simulink model "Test2Part3"  (R2024a)
settings: Solver=VariableStepDiscrete  StartTime=0.0  StopTime=1000  MaxStep=1  RelTol=1e-3
libraries: matrix_library x3
settings Model: Creator=katutu  LastModifiedBy=katutu

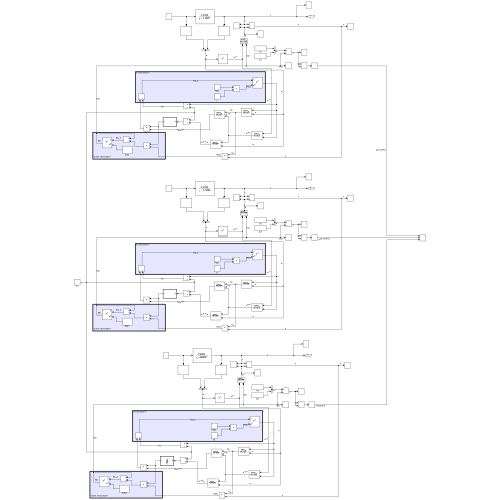
[thumbnail: Simulink's stored preview of the top-level diagram]
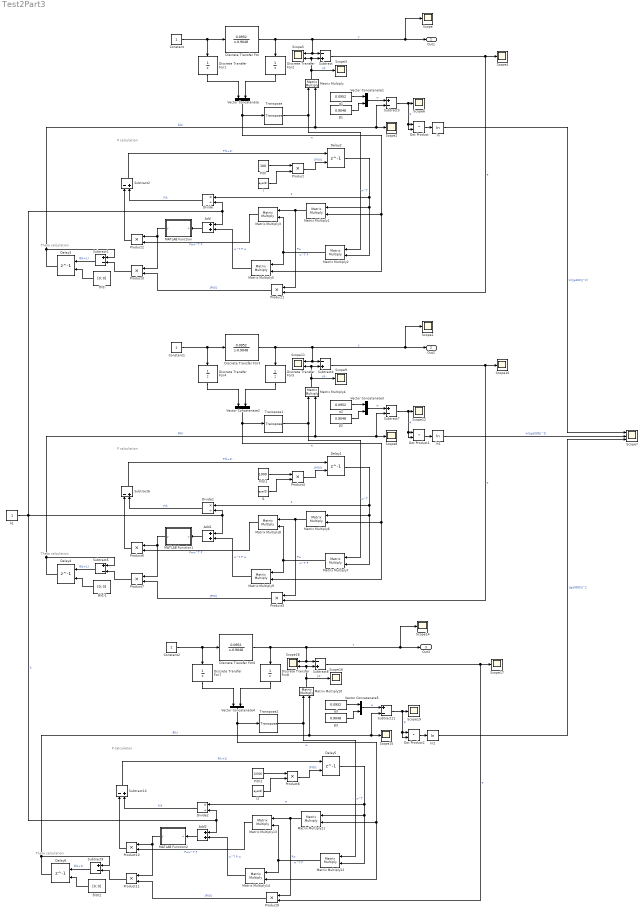
== system Test2Part3 ==
  note: P calculation
  note: Theta calculation
  note: Theta calculation
  note: P calculation
  note: Theta calculation
  note: P calculation
  Add : Sum
  Add1 : Sum
  Add2 : Sum
  Constant : Constant
  Constant1 : Constant
  Constant2 : Constant
  Delay{1..6} (6 alike) : Delay  DelayLength=1  InitialConditionSource=Input port  InitialCondition=0
      settings: InputPortMap=u0,p4
  Discrete Transfer Fcn : DiscreteTransferFcn  Numerator=[0.0952]  Denominator=[1 -0.9048]
  Discrete Transfer Fcn{1..2,4..5,7..8} (6 alike) : DiscreteTransferFcn  Denominator=[1 0]
  Discrete Transfer Fcn3 : DiscreteTransferFcn  Numerator=[0.0952]  Denominator=[1 -0.9048]
  Discrete Transfer Fcn6 : DiscreteTransferFcn  Numerator=[0.0952]  Denominator=[1 -0.9048]
  Divide : Product  Inputs=*/
  Divide1 : Product  Inputs=*/
  Divide2 : Product  Inputs=*/
  Dot Product : DotProduct  OutDataTypeStr=Inherit: Inherit via internal rule
  Dot Product1 : DotProduct  OutDataTypeStr=Inherit: Inherit via internal rule
  Dot Product2 : DotProduct  OutDataTypeStr=Inherit: Inherit via internal rule
  I : Constant  Value=eye(2)
  I1 : Constant  Value=eye(2)
  I2 : Constant  Value=eye(2)
  MATLAB Function : MATLAB Function  TreatAsAtomicUnit=on
  MATLAB Function1 : MATLAB Function  TreatAsAtomicUnit=on
  MATLAB Function2 : MATLAB Function  TreatAsAtomicUnit=on
  Matrix Multiply{,1..14} (15 alike) : Product  Multiplication=Matrix(*)
  P(0) : Constant  Value=100
  P(0)1 : Constant  Value=1000
  P(0)2 : Constant  Value=10000
  Product{,1..11} (12 alike) : Product
  Scope{,1..4,6,8..10,12,14..17,19} (15 alike) : Scope
  Scope11 : Scope  NumInputPorts=2
  Scope18 : Scope  NumInputPorts=2
  Scope5 : Scope  NumInputPorts=2
  Scope7 : Scope  NumInputPorts=3
  Subtract{,2,4,6,8,10} (6 alike) : Sum  Inputs=-+
  Subtract{1,3,5,7,9,11} (6 alike) : Sum  Inputs=+-
  Transpose : matrix_library/Transpose
  Transpose1 : matrix_library/Transpose
  Transpose2 : matrix_library/Transpose
  Vector Concatenate{,1..5} (6 alike) : Concatenate
  ln : Math  Operator=log
  ln1 : Math  Operator=log
  ln2 : Math  Operator=log
  α1 : Constant  Value=0.0952
  α2 : Constant  Value=0.0952
  α3 : Constant  Value=0.0952
  β1 : Constant  Value=0.9048
  β2 : Constant  Value=0.9048
  β3 : Constant  Value=0.9048
  θ(0) : Constant  Value=[0; 0]
  θ(0)1 : Constant  Value=[0; 0]
  θ(0)2 : Constant  Value=[0; 0]
  λ1 : Constant
  Out1 : Outport  SignalName=y
  Out2 : Outport  Port=2  SignalName=y
  Out3 : Outport  Port=3  SignalName=y
  wires:
  Constant/1 -> Discrete Transfer Fcn1/1, Discrete Transfer Fcn/1
  Discrete Transfer Fcn2/1 -> Vector Concatenate/2
  Discrete Transfer Fcn1/1 -> Vector Concatenate/1
  Vector Concatenate/1 -> Matrix Multiply5/2, Matrix Multiply1/2, Transpose/1  "w"
  Matrix Multiply/1 -> Subtract/2, Scope5/2, Scope3/1  "yp"
  Subtract/1 -> Scope4/1, Product1/2  "e"
  Transpose/1 -> Matrix Multiply2/1, Matrix Multiply/1  "w^T"
  Delay3/1 -> Matrix Multiply/2, Subtract3/2, Scope2/1, Subtract1/1  "θ(k)"
  Discrete Transfer Fcn/1 -> Out1/1, Scope/1, Scope5/1, Subtract/1, Discrete Transfer Fcn2/1  "y"
  λ1/1 -> Divide/2, Add/1, Add1/1, Divide1/2, Divide2/2, Add2/1  "λ"
  Delay2/1 -> Divide/1, Matrix Multiply2/2, Matrix Multiply1/1  "P"
  I/1 -> Product/2
  Product/1 -> Delay2/2  "[P(0)]"
  Matrix Multiply1/1 -> Product1/1, Matrix Multiply3/1  "Pw"
  Matrix Multiply2/1 -> Matrix Multiply3/2, Matrix Multiply5/1  "w^T P"
  Matrix Multiply3/1 -> Product2/2  "Pww^T P"
  MATLAB Function/1(y) -> Product3/1, Product2/1
  Add/1 -> MATLAB Function/1(u)
  Matrix Multiply5/1 -> Add/2  "w^T P w"
  P(0)/1 -> Product/1
  Divide/1 -> Subtract2/2  "P/λ"
  Product2/1 -> Subtract2/1
  Subtract2/1 -> Delay2/1  "P(k+1)"
  θ(0)/1 -> Delay3/2
  Subtract1/1 -> Delay3/1  "θ(k+1)"
  Product1/1 -> Product3/2  "[P(0)]"
  Product3/1 -> Subtract1/2
  α1/1 -> Vector Concatenate1/1
  β1/1 -> Vector Concatenate1/2
  Vector Concatenate1/1 -> Subtract3/1  "w"
  Subtract3/1 -> Dot Product/2, Dot Product/1, Scope6/1  "φ"
  Dot Product/1 -> ln/1
  ln/1 -> Scope7/1  "ln(||φ100||^2)"
  Discrete Transfer Fcn3/1 -> Out2/1, Scope1/1, Scope11/1, Subtract4/1, Discrete Transfer Fcn5/1  "y"
  I1/1 -> Product4/2
  Vector Concatenate2/1 -> Matrix Multiply9/2, Matrix Multiply6/2, Transpose1/1  "w"
  Product4/1 -> Delay1/2  "[P(0)]"
  Discrete Transfer Fcn4/1 -> Vector Concatenate2/1
  Delay4/1 -> Matrix Multiply4/2, Subtract7/2, Scope8/1, Subtract5/1  "θ(k)"
  Delay1/1 -> Divide1/1, Matrix Multiply7/2, Matrix Multiply6/1  "P"
  MATLAB Function1/1(y) -> Product7/1, Product6/1
  Matrix Multiply6/1 -> Product5/1, Matrix Multiply8/1  "Pw"
  θ(0)1/1 -> Delay4/2
  Matrix Multiply4/1 -> Subtract4/2, Scope11/2, Scope9/1  "yp"
  Transpose1/1 -> Matrix Multiply7/1, Matrix Multiply4/1  "w^T"
  Subtract7/1 -> Dot Product1/2, Dot Product1/1, Scope12/1  "φ"
  Matrix Multiply7/1 -> Matrix Multiply8/2, Matrix Multiply9/1  "w^T P"
  Product7/1 -> Subtract5/2
  Constant1/1 -> Discrete Transfer Fcn4/1, Discrete Transfer Fcn3/1
  Vector Concatenate3/1 -> Subtract7/1  "w"
  Discrete Transfer Fcn5/1 -> Vector Concatenate2/2
  Add1/1 -> MATLAB Function1/1(u)
  P(0)1/1 -> Product4/1
  Matrix Multiply9/1 -> Add1/2  "w^T P w"
  Product5/1 -> Product7/2  "[P(0)]"
  Matrix Multiply8/1 -> Product6/2  "Pww^T P"
  Subtract6/1 -> Delay1/1  "P(k+1)"
  Subtract5/1 -> Delay4/1  "θ(k+1)"
  β2/1 -> Vector Concatenate3/2
  Subtract4/1 -> Scope10/1, Product5/2  "e"
  ln1/1 -> Scope7/2  "ln(||φ1000||^2)"
  α2/1 -> Vector Concatenate3/1
  Product6/1 -> Subtract6/1
  Divide1/1 -> Subtract6/2  "P/λ"
  Dot Product1/1 -> ln1/1
  Discrete Transfer Fcn6/1 -> Out3/1, Scope14/1, Scope18/1, Subtract8/1, Discrete Transfer Fcn8/1  "y"
  I2/1 -> Product8/2
  Vector Concatenate4/1 -> Matrix Multiply14/2, Matrix Multiply11/2, Transpose2/1  "w"
  Product8/1 -> Delay5/2  "[P(0)]"
  Discrete Transfer Fcn7/1 -> Vector Concatenate4/1
  Delay6/1 -> Matrix Multiply10/2, Subtract11/2, Scope15/1, Subtract9/1  "θ(k)"
  Delay5/1 -> Divide2/1, Matrix Multiply12/2, Matrix Multiply11/1  "P"
  MATLAB Function2/1(y) -> Product11/1, Product10/1
  Matrix Multiply11/1 -> Product9/1, Matrix Multiply13/1  "Pw"
  θ(0)2/1 -> Delay6/2
  Matrix Multiply10/1 -> Subtract8/2, Scope18/2, Scope16/1  "yp"
  Transpose2/1 -> Matrix Multiply12/1, Matrix Multiply10/1  "w^T"
  Subtract11/1 -> Dot Product2/2, Dot Product2/1, Scope19/1  "φ"
  Matrix Multiply12/1 -> Matrix Multiply13/2, Matrix Multiply14/1  "w^T P"
  Product11/1 -> Subtract9/2
  Constant2/1 -> Discrete Transfer Fcn7/1, Discrete Transfer Fcn6/1
  Vector Concatenate5/1 -> Subtract11/1  "w"
  Discrete Transfer Fcn8/1 -> Vector Concatenate4/2
  Add2/1 -> MATLAB Function2/1(u)
  P(0)2/1 -> Product8/1
  Matrix Multiply14/1 -> Add2/2  "w^T P w"
  Product9/1 -> Product11/2  "[P(0)]"
  Matrix Multiply13/1 -> Product10/2  "Pww^T P"
  Subtract10/1 -> Delay5/1  "P(k+1)"
  Subtract9/1 -> Delay6/1  "θ(k+1)"
  β3/1 -> Vector Concatenate5/2
  Subtract8/1 -> Scope17/1, Product9/2  "e"
  ln2/1 -> Scope7/3  "||φ10000||^2"
  α3/1 -> Vector Concatenate5/1
  Product10/1 -> Subtract10/1
  Divide2/1 -> Subtract10/2  "P/λ"
  Dot Product2/1 -> ln2/1

== matlab function Test2Part3/MATLAB Function ==
  data: u input; y output
function y = fcn(u)

y = inv(u);

== matlab function Test2Part3/MATLAB Function2 ==
  data: u input; y output
function y = fcn(u)

y = inv(u);

== matlab function Test2Part3/MATLAB Function1 ==
  data: u input; y output
function y = fcn(u)

y = inv(u);
